simulink model "helix_trajectory_test_data"  (R2021b)
settings: Solver=VariableStepAuto  StartTime=0.0  StopTime=10.0  RelTol=1e-3
settings Model: Creator=HP Owner  LastModifiedBy=HP Owner

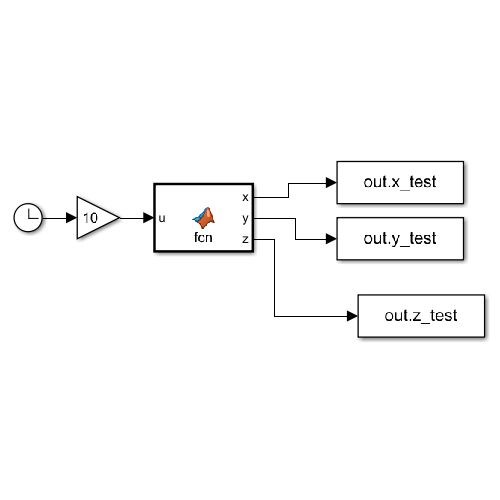
[thumbnail: Simulink's stored preview of the top-level diagram]
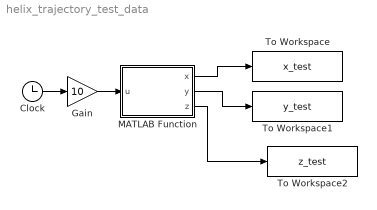
== system helix_trajectory_test_data ==
  Clock : Clock
  Gain : Gain  Gain=10
  MATLAB Function : MATLAB Function  TreatAsAtomicUnit=on
  To Workspace : ToWorkspace  VariableName=x_test  SampleTime=-1
  To Workspace1 : ToWorkspace  VariableName=y_test  SampleTime=-1
  To Workspace2 : ToWorkspace  VariableName=z_test  SampleTime=-1
  wires:
  Clock/1 -> Gain/1
  MATLAB Function/1(x) -> To Workspace/1
  MATLAB Function/2(y) -> To Workspace1/1
  MATLAB Function/3(z) -> To Workspace2/1
  Gain/1 -> MATLAB Function/1(u)

== matlab function helix_trajectory_test_data/MATLAB Function ==
  data: x output; u input; y output; z output
function [x,y,z] = fcn(u)
x = sind(u)*cosd(20*u);
y = sind(u)*sind(20*u);
z = cosd(u);
